simulink model "astrobotics_flowchart1"  (R2017a)
settings: Solver=FixedStepDiscrete  StartTime=0.0  StopTime=60  FixedStep=0.1  RelTol=1e-3  EnableMultiTasking=on
settings Model: Creator=alex  LastModifiedBy=alex
settings SolverCC: AutoInsertRateTranBlk=on
settings DataIOCC: LimitDataPoints=on
settings OptimizationCC: LifeSpan=inf
settings DebuggingCC: AllowSymbolicDim=off  SFUnexpectedBacktrackingDiag=warning  SFNoUnconditionalDefaultTransitionDiag=warning  SFExecutionAtInitializationDiag=none
settings GRTTargetCC: TargetLangStandard=C89/C90 (ANSI)
settings ConfigComp: CovMetricSettings=dw  CovHtmlReporting=on  CovSaveCumulativeToWorkspaceVar=on  CovSaveSingleToWorkspaceVar=on  CovShowResultsExplorer=off  CovExternalEMLEnable=off

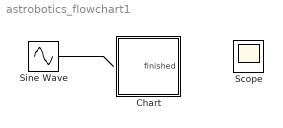
== system astrobotics_flowchart1 ==
  Chart : Stateflow chart  TreatAsAtomicUnit=on
  Scope : Scope
  Sine Wave : Sin  SampleTime=0
  wires:
  Sine Wave/1 -> ?
  ? -> Scope/1

== stateflow chart astrobotics_flowchart1/Chart ==
  state start
    entry: state_select = 0;
    state_select = state_select + 1;
    cycles = 0;
    finished = false;
  state deposit_material
    entry: state_select = 4;
    cycles = cycles + 1;
    state_select = 1;
    if cycles == 5
    state_select = 5;
    end
  state drive_out %State Name
    entry: state_select = 1; % entry action
    state_select = state_select + 1;
    % during:
  state excavate
    entry: state_select = 2;
    state_select = state_select + 1;
  state drive_in
    entry: state_select = 3;
    state_select = state_select + 1;
  state stop
    entry: state_select = 5;
    finished = true;
  (default) -> start : {state_select = 0;}
  start -> drive_out %State Name : [state_select == 1]
  deposit_material -> stop [order 2] : [state_select == 5]
  deposit_material -> drive_out %State Name [order 1] : [state_select == 1]
  drive_out %State Name -> excavate : [state_select == 2]% [transition condition]{action}
  drive_in -> deposit_material : [state_select ==  4]
  excavate -> drive_in : [state_select == 3]
  data: finished output; cycles local; state_select local int32
